simulink model "example_DataFromFile"  (R2016b)
settings: Solver=ode45  StartTime=0.0  StopTime=365*24*3600  RelTol=1e-3  EnableMultiTasking=on
libraries: carnot x2
settings Model: Creator=drhf  LastModifiedBy=drhf
settings DataIOCC: LimitDataPoints=on  SaveFormat=Array
settings OptimizationCC: ExpressionDepthLimit=2147483647  LifeSpan=inf
settings DebuggingCC: UnderspecifiedInitializationDetection=Classic  MergeDetectMultiDrivingBlocksExec=none  SolverPrmCheckMsg=warning  StateNameClashWarn=warning  SFUnexpectedBacktrackingDiag=warning  SFNoUnconditionalDefaultTransitionDiag=warning  SFExecutionAtInitializationDiag=none
settings HardwareCC: ProdBitPerPointer=32  ProdBitPerSizeT=32  ProdBitPerPtrDiffT=32  ProdLargestAtomicFloat=None  ProdIntDivRoundTo=Undefined  ProdEndianess=Unspecified  ProdWordSize=32  ProdHWDeviceType=32-bit Generic
settings ModelReferenceCC: PropagateSignalLabelsOutOfModel=off
settings GRTTargetCC: TargetLangStandard=C89/C90 (ANSI)  GeneratePreprocessorConditionals=Disable all  CombineOutputUpdateFcns=off  GRTInterface=on
settings ConfigComp: CovMetricSettings=dw  CovHtmlReporting=on  CovSaveCumulativeToWorkspaceVar=on  CovSaveSingleToWorkspaceVar=on  CovExternalEMLEnable=off

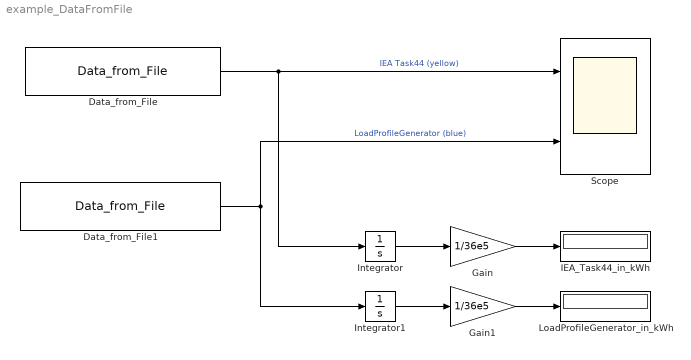
== system example_DataFromFile ==
  Data_from_File : carnot/Load/General/Data_from_File  PathName='C:\repos\carnot_svn\trunk\public\data\'  FileName='ElectricProfile_SHC_IEA_Task44.mat'  UserParam=off  VariableName=ElectricProfile_SHC_IEA_Task44  SampleTime=60
  Data_from_File1 : carnot/Load/General/Data_from_File  PathName='C:\repos\carnot_svn\trunk\public\data\'  FileName='ElectricProfile_loadprofilegenerator.mat'  UserParam=off  VariableName=ElectricProfile_loadprofilegenerator  SampleTime=60
  Gain : Gain  Gain=1/36e5
  Gain1 : Gain  Gain=1/36e5
  IEA_Task44_in_kWh : Display
  Integrator : Integrator
  Integrator1 : Integrator
  LoadProfileGenerator_in_kWh : Display
  Scope : Scope  NumInputPorts=2
  wires:
  Data_from_File/1 -> Integrator/1, Scope/1  "IEA Task44 (yellow)"
  Data_from_File1/1 -> Scope/2, Integrator1/1  "LoadProfileGenerator (blue)"
  Integrator/1 -> Gain/1
  Integrator1/1 -> Gain1/1
  Gain/1 -> IEA_Task44_in_kWh/1
  Gain1/1 -> LoadProfileGenerator_in_kWh/1
